simulink model "subsistema_electromagnetico"  (R2023b)
settings: Solver=VariableStepAuto  StartTime=0.0  StopTime=10.0  RelTol=1e-3
values from neighbouring files (symbols this model uses):
  L_d = 6.6e-3    (= 0.0066)    [controlador_foc_simulink.m]    (also in params_subsistema_electromagnetico.m; sistema_completo_en_codigo.m)
  L_l = 0.8e-3    (= 0.0008)    [controlador_foc_simulink.m]    (also in params_subsistema_electromagnetico.m; sistema_completo_en_codigo.m)
  L_q = 5.8e-3    (= 0.0058)    [controlador_foc_simulink.m]    (also in params_subsistema_electromagnetico.m; sistema_completo_en_codigo.m)
  lambda_m = 0.016    [controlador_foc_simulink.m]    (also in parametros_planta.m; params_subsistema_electromagnetico.m; sistema_completo_en_codigo.m)
  Pp = 3    [controlador_foc_simulink.m]    (also in parametros_planta.m; params_subsistema_electromagnetico.m; sistema_completo_en_codigo.m)
settings Model: Creator=Pc  LastModifiedBy=Pc

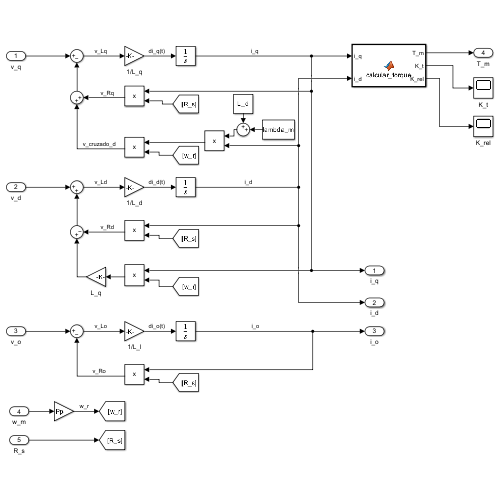
[thumbnail: Simulink's stored preview of the top-level diagram]
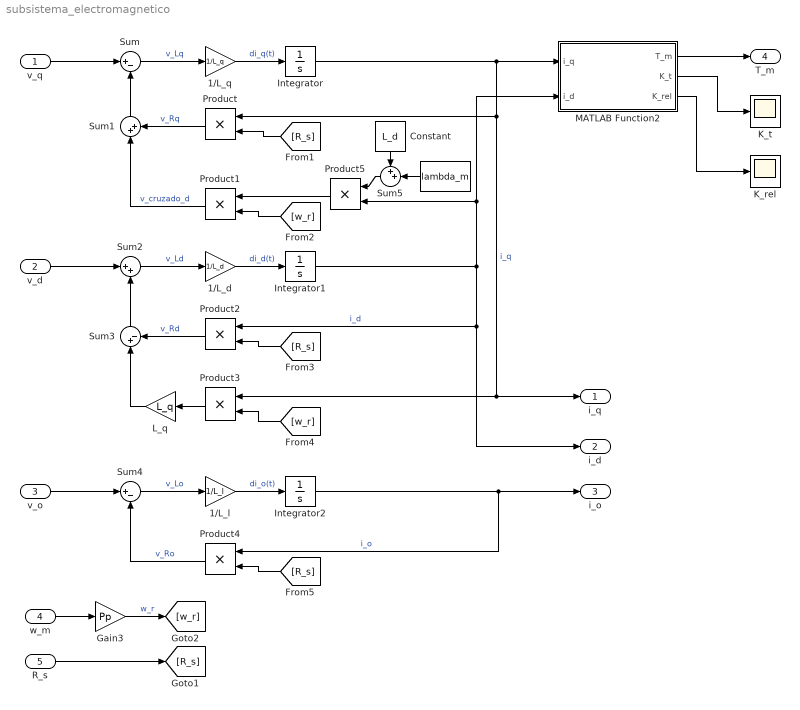
== system subsistema_electromagnetico ==
  v_q : Inport
  v_d : Inport  Port=2
  v_o : Inport  Port=3
  w_m : Inport  Port=4
  R_s : Inport  Port=5
  " " : Constant  Value=lambda_m
  1/L_d : Gain  Gain=1/L_d
  1/L_l : Gain  Gain=1/L_l
  1/L_q : Gain  Gain=1/L_q
  Constant : Constant  Value=L_d
  Gain3 : Gain  Gain=Pp
  Integrator : Integrator
  Integrator1 : Integrator
  Integrator2 : Integrator
  K_rel : Scope
  K_t : Scope
  L_q : Gain  Gain=L_q
  MATLAB Function2 : MATLAB Function  TreatAsAtomicUnit=on
  Product{,1..5} (6 alike) : Product
  Sum : Sum  Inputs=|+-
  Sum1 : Sum  Inputs=|++
  Sum2 : Sum  Inputs=|++
  Sum3 : Sum  Inputs=|+-
  Sum4 : Sum  Inputs=|+-
  Sum5 : Sum  Inputs=++|
  i_q : Outport
  i_d : Outport  Port=2
  i_o : Outport  Port=3
  T_m : Outport  Port=4
  wires:
  L_q/1 -> Sum3/1
  Gain3/1 -> [w_r]  "w_r"
  1/L_l/1 -> Integrator2/1  "di_o(t)"
  Integrator1/1 -> MATLAB Function2/2(i_d), Product5/2, i_d/1, Product2/1  "i_d"
  R_s/1 -> [R_s]
  MATLAB Function2/2(K_t) -> K_t/1
  Sum5/1 -> Product5/1
  MATLAB Function2/1(T_m) -> T_m/1
  " "/1 -> Sum5/2
  [w_r] -> Product1/2
  w_m/1 -> Gain3/1
  Sum4/1 -> 1/L_l/1  "v_Lo"
  v_o/1 -> Sum4/1
  MATLAB Function2/3(K_rel) -> K_rel/1
  Sum/1 -> 1/L_q/1  "v_Lq"
  Product4/1 -> Sum4/2  "v_Ro"
  [R_s] -> Product2/2
  v_q/1 -> Sum/1
  v_d/1 -> Sum2/1
  Product/1 -> Sum1/2  "v_Rq"
  [R_s] -> Product/2
  1/L_q/1 -> Integrator/1  "di_q(t)"
  [w_r] -> Product3/2
  Product2/1 -> Sum3/2  "v_Rd"
  Sum1/1 -> Sum/2
  Product1/1 -> Sum1/1  "v_cruzado_d"
  Integrator2/1 -> i_o/1, Product4/1  "i_o"
  Sum3/1 -> Sum2/2
  Integrator/1 -> MATLAB Function2/1(i_q), Product/1, i_q/1, Product3/1  "i_q"
  [R_s] -> Product4/2
  1/L_d/1 -> Integrator1/1  "di_d(t)"
  Product5/1 -> Product1/1
  Product3/1 -> L_q/1
  Constant/1 -> Sum5/1
  Sum2/1 -> 1/L_d/1  "v_Ld"

== matlab function subsistema_electromagnetico/MATLAB Function2 ==
  data: i_q input; i_d input; T_m output; Pp parameter; lambda_m parameter; L_d parameter; L_q parameter; K_t output; K_rel output
function [T_m, K_t, K_rel] = calcular_torque(i_q, i_d, Pp, lambda_m, L_d, L_q)
    % CALCULAR_TORQUE Calcula el torque electromagnético total de la máquina PMSM
    % y sus constantes equivalentes.
    % 
    % Entradas dinámicas (Inports):
    %   i_q      : Corriente en el eje en cuadratura [A].
    %   i_d      : Corriente en el eje directo [A].
    %
    % Parámetros estáticos (Parameters):
    %   P_p      : Número de pares de polos.
    %   lambda_m : Flujo magnético de los imanes permanentes [Wb].
    %   L_d      : Inductancia del eje d [H].
    %   L_q      : Inductancia del eje q [H].
    %
    % Salidas:
    %   T_m      : Torque electromagnético generado [N.m].
    %   K_t      : Constante de torque de alineación [N.m/A].
    %   K_rel    : Constante de torque de reluctancia [N.m/A^2].

    % 1. Cálculo de las constantes 
    K_t = (3/2) * Pp * lambda_m;
    K_rel = (3/2) * Pp * (L_d - L_q);

    % 2. Cálculo del torque electromagnético total
    T_m = K_t * i_q + K_rel * i_d * i_q;
end
